simulink model "mech_gears_backlash"  (Simulink 7.1)
settings: Solver=ode23tb  StartTime=0.0  StopTime=20
InitFcn:
  | gear.backlashCW=0.2;
  | gear.backlashCCW=0.2;
undefined symbols (not defined in the file or in its folder): rad, s
libraries: mblibv1 x19, simulink x1
Description:
  | Gears with Backlash
  | 
  | Two gears with forward actuation and intergear backlash. Gear radius ratio: GearB:GearA is 1:3.
settings Model: Creator=arnav  LastModifiedBy=batserve  ExtModeAutoUpdateStatusClock=off
settings DataIOCC: OutputOption=SpecifiedOutputTimes  OutputTimes=linspace(0,20,300)  Refine=5
settings OptimizationCC: InlineInvariantSignals=on
settings DebuggingCC: SaveWithParameterizedLinksMsg=none  SignalResolutionControl=TryResolveAllWithWarning  SolverPrmCheckMsg=none  MultiTaskDSMMsg=warning  MultiTaskCondExecSysMsg=none  SigSpecEnsureSampleTimeMsg=none  StrictBusMsg=None
settings HardwareCC: TargetBitPerLong=64  TargetEndianess=LittleEndian  TargetWordSize=64  TargetHWDeviceType=MATLAB Host  ProdEqTarget=off
settings RTWCC: SystemTargetFile=rsim.tlc  TemplateMakefile=rsim_default_tmf  Description=Rapid Simulation Target  ProcessScript=rsim_make_rtw_hook  IncludeERTFirstTime=on
settings RSimTargetCC: TargetFcnLib=ansi_tfl_tmw.mat  TargetFunctionLibrary=ANSI_C  IsPILTarget=off  EnableShiftOperators=on  PortableWordSizes=off
settings SimMechanicsCC: VisOnUpdateDiagram=on  VisDuringSimulation=on  VisConfigFile=mech_gears_backlash.mat

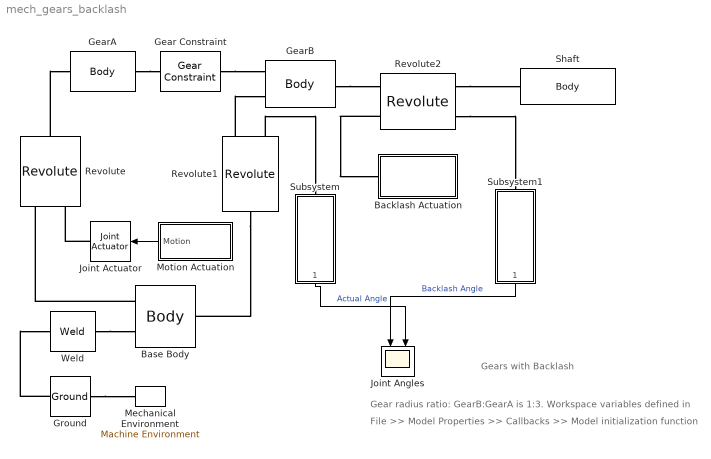
== system mech_gears_backlash ==
  note: Gears with Backlash
  note: Gear radius ratio: GearB:GearA is 1:3.
      | Workspace variables defined in
  note: File >> Model Properties >>
      | Callbacks >> Model initialization function
  Backlash Actuation : Subsystem
  Base Body : mblibv1/Bodies/Body  DialogController=MECH.DynMechDlgSource  PhysicalDomain=mechanical  SubClassName=Unknown  LeftPortType=workingframe  RightPortType=workingframe  LConnTagsString=CS1|CG  RConnTagsString=CS2  DialogClass=MechanicalBodyBlock  Mass=14  MassUnits=kg  InertiaUnits=kg*m^2  Inertia=[1 0 0;0 3 0;0 0 3];  Shape=Cylinder  ShapeDims=[1 1]  ShapeUnits=m  ShapeUse=false  Density=1  DensityUnits=kg/m^3  DensityUse=false  GraphicsMode=1  BodyColor=[0.5 0.5 0.5]  GraphicsObj=[]  AttachedToCS=1  CG=Left$CG$[1 0 0]$CS1$CS1$m$[0 0 0]$Euler X-Y-Z$deg$WORLD$true  WorkingFrames=Left$CS1$[0 0 0]$WORLD$WORLD$m$[0 0 0]$Euler X-Y-Z$deg$WORLD$true#Right$CS2$[2 0 0]$CS1$CS1$m$[0 0 0]$Euler X-Y-Z$deg$WORLD$true#Right$CS3$[1 -2 0]$CS1$CS1$m$[0 0 0]$Euler X-Y-Z$deg$WORLD$false  CGPos=[1 0 0]  CGRot=[0 0 0]  CS0Pos=[]  CS0Rot=[]  CS1Pos=[0 0 0]  CS1Rot=[0 0 0]  CS2Pos=[2 0 0]  CS2Rot=[0 0 0]  CS3Pos=[1 -2 0]  CS3Rot=[0 0 0]  CS4Pos=[]  CS4Rot=[]  CS5Pos=[]  CS5Rot=[]  CS6Pos=[]  CS6Rot=[]  CS7Pos=[]  CS7Rot=[]  CS8Pos=[]  CS8Rot=[]  CS9Pos=[]  CS9Rot=[]  CS10Pos=[]  CS10Rot=[]  CS11Pos=[]  CS11Rot=[]  CS12Pos=[]  CS12Rot=[]  CS13Pos=[]  CS13Rot=[]  CS14Pos=[]  CS14Rot=[]  CS15Pos=[]  CS15Rot=[]  CS16Pos=[]  CS16Rot=[]  CS17Pos=[]  CS17Rot=[]  CS18Pos=[]  CS18Rot=[]  CS19Pos=[]  CS19Rot=[]  CS20Pos=[]  CS20Rot=[]
  Gear Constraint : mblibv1/Constraints &  Drivers/Gear Constraint  DialogController=MECH.DynMechDlgSource  PhysicalDomain=mechanical  SubClassName=Unknown  LeftPortType=blob  RightPortType=blob  LConnTagsString=__newl0  RConnTagsString=__newr0  DialogClass=GearConstraint  NumSAPorts=0  BaseRadius=1.5  BaseRadiusUnits=m  FollowerRadius=0.5  FollowerRadiusUnits=m
  GearA : mblibv1/Bodies/Body  DialogController=MECH.DynMechDlgSource  PhysicalDomain=mechanical  SubClassName=Unknown  LeftPortType=workingframe  RightPortType=workingframe  LConnTagsString=CS1  RConnTagsString=CS2  DialogClass=MechanicalBodyBlock  Mass=2  MassUnits=kg  InertiaUnits=kg*m^2  Inertia=[0.5 0 0;0 0.5 0;0 0 1]  Shape=Cylinder  ShapeDims=[1 1]  ShapeUnits=m  ShapeUse=false  Density=1  DensityUnits=kg/m^3  DensityUse=false  GraphicsMode=1  BodyColor=[0.5 0.5 0.5]  GraphicsObj=[]  AttachedToCS=1  CG=Left$CG$[0 0 0]$CS1$CS1$m$[0 0 0]$Euler X-Y-Z$deg$WORLD$false  WorkingFrames=Left$CS1$[0 0 0]$ADJOINING$ADJOINING$m$[0 0 0]$Euler X-Y-Z$deg$WORLD$true#Right$CS2$[0 0 0]$CS1$CS1$m$[0 0 0]$Euler X-Y-Z$deg$WORLD$true#Right$CS3$[-1 0 0]$CG$CG$m$[0 0 0]$Euler X-Y-Z$deg$WORLD$false#Right$CS4$[0 1 0]$CG$CG$m$[0 0 0]$Euler X-Y-Z$deg$WORLD$false#Right$CS5$[1 0 0]$CG$CG$m$[0 0 0]$Euler X-Y-Z$deg$WORLD$false#Right$CS6$[0 -1 0]$CG$CG$m$[0 0 0]$Euler X-Y-Z$deg$WORLD$false#Right$CS7$[0 0 -0.5]$CS3$CS3$m$[0 0 0]$Euler X-Y-Z$deg$WORLD$false#Right$CS8$[0 0 -0.5]$CS4$CS4$m$[0 0 0]$Euler X-Y-Z$deg$WORLD$false#Right$CS9$[0 0 -0.5]$CS5$CS5$m$[0 0 0]$Euler X-Y-Z$deg$WORLD$false#Right$CS10$[0 0 -0.5]$CS6$CS6$m$[0 0 0]$Euler X-Y-Z$deg$WORLD$false  CGPos=[0 0 0]  CGRot=[0 0 0]  CS0Pos=[]  CS0Rot=[]  CS1Pos=[0 0 0]  CS1Rot=[0 0 0]  CS2Pos=[0 0 0]  CS2Rot=[0 0 0]  CS3Pos=[-1 0 0]  CS3Rot=[0 0 0]  CS4Pos=[0 1 0]  CS4Rot=[0 0 0]  CS5Pos=[1 0 0]  CS5Rot=[0 0 0]  CS6Pos=[0 -1 0]  CS6Rot=[0 0 0]  CS7Pos=[0 0 -0.5]  CS7Rot=[0 0 0]  CS8Pos=[0 0 -0.5]  CS8Rot=[0 0 0]  CS9Pos=[0 0 -0.5]  CS9Rot=[0 0 0]  CS10Pos=[0 0 -0.5]  CS10Rot=[0 0 0]  CS11Pos=[]  CS11Rot=[]  CS12Pos=[]  CS12Rot=[]  CS13Pos=[]  CS13Rot=[]  CS14Pos=[]  CS14Rot=[]  CS15Pos=[]  CS15Rot=[]  CS16Pos=[]  CS16Rot=[]  CS17Pos=[]  CS17Rot=[]  CS18Pos=[]  CS18Rot=[]  CS19Pos=[]  CS19Rot=[]  CS20Pos=[]  CS20Rot=[]
  GearB : mblibv1/Bodies/Body  DialogController=MECH.DynMechDlgSource  PhysicalDomain=mechanical  SubClassName=Unknown  LeftPortType=workingframe  RightPortType=workingframe  LConnTagsString=CS1|CS2  RConnTagsString=CS3  DialogClass=MechanicalBodyBlock  Mass=4  MassUnits=kg  InertiaUnits=kg*m^2  Inertia=[0.5 0 0;0 0.5 0;0 0 1]  Shape=Cylinder  ShapeDims=[1 1]  ShapeUnits=m  ShapeUse=false  Density=1  DensityUnits=kg/m^3  DensityUse=false  GraphicsMode=1  BodyColor=[0.5 0.5 0.5]  GraphicsObj=[]  AttachedToCS=1  CG=Left$CG$[0 0 0]$CS1$CS1$m$[0 0 0]$Euler X-Y-Z$deg$WORLD$false  WorkingFrames=Left$CS1$[2 0 0]$ADJOINING$ADJOINING$m$[0 0 0]$Euler X-Y-Z$deg$WORLD$true#Left$CS2$[0 0 0]$CS1$CS1$m$[0 0 0]$Euler X-Y-Z$deg$WORLD$true#Right$CS3$[0 0 0]$CS1$CS1$m$[0 0 0]$Euler X-Y-Z$deg$WORLD$true#Right$CS4$[1 0 0]$CG$CG$m$[0 0 0]$Euler X-Y-Z$deg$WORLD$false#Right$CS5$[0 1 0]$CG$CG$m$[0 0 0]$Euler X-Y-Z$deg$WORLD$false#Right$CS6$[-1 0 0]$CG$CG$m$[0 0 0]$Euler X-Y-Z$deg$WORLD$false#Right$CS7$[0 -1 0]$CG$CG$m$[0 0 0]$Euler X-Y-Z$deg$WORLD$false#Right$CS8$[0 0 -0.5]$CS4$CS4$m$[0 0 0]$Euler X-Y-Z$deg$WORLD$false#Right$CS9$[0 0 -0.5]$CS5$CS5$m$[0 0 0]$Euler X-Y-Z$deg$WORLD$false#Right$CS10$[0 0 -0.5]$CS6$CS6$m$[0 0 0]$Euler X-Y-Z$deg$WORLD$false#Right$CS11$[0 0 -0.5]$CS7$CS7$m$[0 0 0]$Euler X-Y-Z$deg$WORLD$false  CGPos=[0 0 0]  CGRot=[0 0 0]  CS0Pos=[]  CS0Rot=[]  CS1Pos=[2 0 0]  CS1Rot=[0 0 0]  CS2Pos=[0 0 0]  CS2Rot=[0 0 0]  CS3Pos=[0 0 0]  CS3Rot=[0 0 0]  CS4Pos=[1 0 0]  CS4Rot=[0 0 0]  CS5Pos=[0 1 0]  CS5Rot=[0 0 0]  CS6Pos=[-1 0 0]  CS6Rot=[0 0 0]  CS7Pos=[0 -1 0]  CS7Rot=[0 0 0]  CS8Pos=[0 0 -0.5]  CS8Rot=[0 0 0]  CS9Pos=[0 0 -0.5]  CS9Rot=[0 0 0]  CS10Pos=[0 0 -0.5]  CS10Rot=[0 0 0]  CS11Pos=[0 0 -0.5]  CS11Rot=[0 0 0]  CS12Pos=[]  CS12Rot=[]  CS13Pos=[]  CS13Rot=[]  CS14Pos=[]  CS14Rot=[]  CS15Pos=[]  CS15Rot=[]  CS16Pos=[]  CS16Rot=[]  CS17Pos=[]  CS17Rot=[]  CS18Pos=[]  CS18Rot=[]  CS19Pos=[]  CS19Rot=[]  CS20Pos=[]  CS20Rot=[]
  Ground : mblibv1/Bodies/Ground  Orientation=left  DialogController=MECH.DynMechDlgSource  SystemSampleTime=-1  LeftPortType=env  RightPortType=workingframe  PhysicalDomain=Mechanical  DialogClass=GroundBlock  CoordPosition=[1 0 0]  CoordPositionUnits=m  StateVectorMgrId=-1  MachineId=[0 0]  ShowEnvPort=on
  Joint Actuator : mblibv1/Sensors &  Actuators/Joint Actuator  Orientation=left  DialogController=MECH.DynMechDlgSource  SystemSampleTime=-1  PhysicalDomain=Mechanical  PortType=blob  ActuationStyle=Motion  AngleUnits=rad  ArcVelocityUnits=rad/s  ArcAccelerationUnits=rad/s^2  CoordPositionUnits=m  VelocityUnits=m/s  AccelerationUnits=m/s^2  ForceUnits=N  TorqueUnits=N-m  ActiveIO=on  Width=3  DialogClass=MechanicalActuatorBlock  Primitive=R1  ReferenceFrame=Absolute (INERTIAL)
  Joint Angles : Scope  NumInputPorts=2
      settings: Orientation=down  TimeRange=20  YMin=-0.25~-2  YMax=0.25~16  SaveName=ScopeData2
  Mechanical Environment : mblibv1/Bodies/Machine Environment  Tag=Factory ground  Orientation=left  DialogController=MECH.DialogSource  SystemSampleTime=-1  PortType=env  PhysicalDomain=Mechanical  DialogTemplateClass=MECH.MachineEnvironment  SyncWhenCopied=off  Gravity=[0 -9.81 0]  GravityUnits=m/s^2  GravityAsSignal=off  Dimensionality=3D Only  AnalysisType=Forward dynamics  LinearAssemblyTolerance=1e-3  LinearAssemblyToleranceUnits=m  AngularAssemblyTolerance=1e-3  AngularAssemblyToleranceUnits=rad  ConstraintSolverType=Stabilizing  ConstraintRelTolerance=1e-4  ConstraintAbsTolerance=1e-4  UseRobustSingularityHandling=off  RedundancyAnalysisToleranceType=Automatically select tolerance  RedundancyAnalysisTolerance=1e-14  StatePerturbationType=Fixed  PerturbationSize=1e-5  VisualizeMachine=on
  Motion Actuation : Subsystem  Orientation=left
  Revolute : mblibv1/Joints/Revolute  Orientation=up  DialogController=MECH.DynMechDlgSource  PhysicalDomain=mechanical  SubClassName=Unknown  LeftPortType=blob  RightPortType=blob  LConnTagsString=__newl0|SA1  RConnTagsString=__newr0  NumSAPorts=1  CutJoint=off  MarkAsCut=off  Primitives=revolute  PrimitiveProps=R1$WORLD$[0 0 1]$revolute  DialogClass=JointBlock  R1Axis=[0 0 1]
  Revolute1 : mblibv1/Joints/Revolute  Orientation=down  DialogController=MECH.DynMechDlgSource  PhysicalDomain=mechanical  SubClassName=Unknown  LeftPortType=blob  RightPortType=blob  LConnTagsString=__newl0|SA1  RConnTagsString=__newr0  NumSAPorts=1  CutJoint=off  MarkAsCut=off  Primitives=revolute  PrimitiveProps=R1$WORLD$[0 0 1]$revolute  DialogClass=JointBlock  R1Axis=[0 0 1]
  Revolute2 : mblibv1/Joints/Revolute  DialogController=MECH.DynMechDlgSource  PhysicalDomain=mechanical  SubClassName=Unknown  LeftPortType=blob  RightPortType=blob  LConnTagsString=__newl0|SA1  RConnTagsString=__newr0|SA1  NumSAPorts=2  CutJoint=off  MarkAsCut=off  Primitives=revolute  PrimitiveProps=R1$WORLD$[0 0 1]$revolute  DialogClass=JointBlock  R1Axis=[0 0 1]
  Shaft : mblibv1/Bodies/Body  DialogController=MECH.DynMechDlgSource  PhysicalDomain=mechanical  SubClassName=Unknown  LeftPortType=workingframe  RightPortType=workingframe  LConnTagsString=CS1  DialogClass=MechanicalBodyBlock  Mass=10  MassUnits=kg  InertiaUnits=kg*m^2  Inertia=[3 0 0;0 3 0;0 0 0.2];  Shape=Cylinder  ShapeDims=[1 1]  ShapeUnits=m  ShapeUse=false  Density=1  DensityUnits=kg/m^3  DensityUse=false  GraphicsMode=1  BodyColor=[0.5 0.5 0.5]  GraphicsObj=[]  AttachedToCS=1  CG=Left$CG$[0 0 1.5]$CS1$CS1$m$[0 0 0]$Euler X-Y-Z$deg$WORLD$false  WorkingFrames=Left$CS1$[0 0 0]$ADJOINING$ADJOINING$m$[0 0 0]$Euler X-Y-Z$deg$WORLD$true#Right$CS2$[0 1.5 0]$CG$CG$m$[0 0 0]$Euler X-Y-Z$deg$WORLD$false#Right$CS3$[0 -1.5 0]$CG$CG$m$[0 0 0]$Euler X-Y-Z$deg$WORLD$false#Right$CS4$[0 0 1]$CS2$CS2$m$[0 0 0]$Euler X-Y-Z$deg$WORLD$false#Right$CS5$[0 0 1]$CS3$CS3$m$[0 0 0]$Euler X-Y-Z$deg$WORLD$false  CGPos=[0 0 1.5]  CGRot=[0 0 0]  CS0Pos=[]  CS0Rot=[]  CS1Pos=[0 0 0]  CS1Rot=[0 0 0]  CS2Pos=[0 1.5 0]  CS2Rot=[0 0 0]  CS3Pos=[0 -1.5 0]  CS3Rot=[0 0 0]  CS4Pos=[0 0 1]  CS4Rot=[0 0 0]  CS5Pos=[0 0 1]  CS5Rot=[0 0 0]  CS6Pos=[]  CS6Rot=[]  CS7Pos=[]  CS7Rot=[]  CS8Pos=[]  CS8Rot=[]  CS9Pos=[]  CS9Rot=[]  CS10Pos=[]  CS10Rot=[]  CS11Pos=[]  CS11Rot=[]  CS12Pos=[]  CS12Rot=[]  CS13Pos=[]  CS13Rot=[]  CS14Pos=[]  CS14Rot=[]  CS15Pos=[]  CS15Rot=[]  CS16Pos=[]  CS16Rot=[]  CS17Pos=[]  CS17Rot=[]  CS18Pos=[]  CS18Rot=[]  CS19Pos=[]  CS19Rot=[]  CS20Pos=[]  CS20Rot=[]
  Subsystem : Subsystem  Orientation=down
  Subsystem1 : Subsystem  Orientation=down
  Weld : mblibv1/Joints/Weld  DialogController=MECH.DynMechDlgSource  PhysicalDomain=mechanical  SubClassName=Unknown  LeftPortType=blob  RightPortType=blob  LConnTagsString=__newl0  RConnTagsString=__newr0  NumSAPorts=0  CutJoint=off  MarkAsCut=off  Primitives=weld  PrimitiveProps=W$INERTIAL$[0 0 0]$weld  DialogClass=JointBlock  WAxis=[0 0 0]
  wires:
  Motion Actuation/1(Motion) -> Joint Actuator/1
  Subsystem1/1(Backlash Angle) -> Joint Angles/1  "Backlash Angle"
  Subsystem/1(Actual Angle) -> Joint Angles/2  "Actual Angle"
  connections:
  Gear Constraint/RConn1 -- GearB/LConn1
  GearA/RConn1 -- Gear Constraint/LConn1
  Ground/LConn1 -- Mechanical Environment/RConn1
  Revolute1/RConn1 -- Base Body/RConn1
  GearB/RConn1 -- Revolute2/LConn1
  Revolute2/RConn1 -- Shaft/LConn1
  Revolute1/LConn1 -- GearB/LConn2
  Ground/RConn1 -- Weld/LConn1
  Weld/RConn1 -- Base Body/LConn2
  Base Body/LConn1 -- Revolute/LConn1
  Revolute/RConn1 -- GearA/LConn1
  Joint Actuator/RConn1 -- Revolute/LConn2
  Revolute2/LConn2 -- Backlash Actuation/LConn1
  Revolute2/RConn2 -- Subsystem1/LConn1
  Revolute1/LConn2 -- Subsystem/LConn1

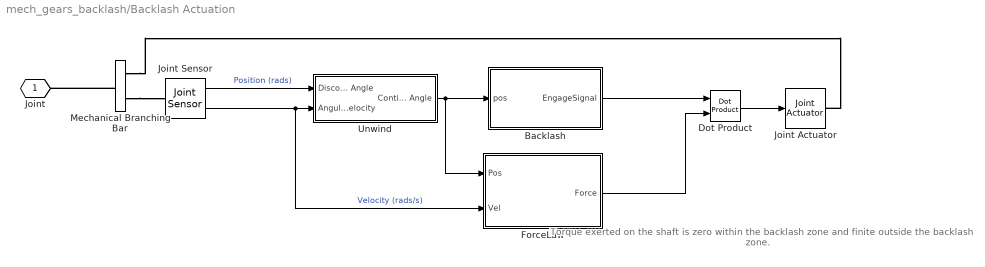
== system mech_gears_backlash/Backlash Actuation ==
  note: Torque exerted on the shaft is zero
      | within the backlash zone and finite
      | outside the backlash zone.
  Backlash : Subsystem
  Dot Product : simulink/Math Operations/Dot Product  InputSameDT=on  OutDataType=sfix(16)  OutScaling=2^-10  DoSatur=off
  ForceLaw : Subsystem
  Joint Actuator : mblibv1/Sensors &  Actuators/Joint Actuator  DialogController=MECH.DynMechDlgSource  SystemSampleTime=-1  PhysicalDomain=Mechanical  PortType=blob  ActuationStyle=Force  AngleUnits=deg  ArcVelocityUnits=deg/s  ArcAccelerationUnits=deg/s^2  CoordPositionUnits=m  VelocityUnits=m/s  AccelerationUnits=m/s^2  ForceUnits=N  TorqueUnits=N-m  ActiveIO=on  Width=1  DialogClass=MechanicalActuatorBlock  Primitive=R1  ReferenceFrame=Absolute (INERTIAL)
  Joint Sensor : mblibv1/Sensors &  Actuators/Joint Sensor  DialogController=MECH.DynMechDlgSource  SystemSampleTime=-1  PhysicalDomain=Mechanical  PortType=blob  Muxed=off  Pose=off  Angle=on  AngleUnits=rad  ArcVelocity=on  ArcVelocityUnits=rad/s  ArcAcceleration=off  ArcAccelerationUnits=deg/s^2  CoordPosition=off  CoordPositionUnits=m  Velocity=off  VelocityUnits=m/s  Acceleration=off  AccelerationUnits=m/s^2  Quaternion=off  QuaternionDT=off  QuaternionDDT=off  QuaternionUnits=off  OutputVector=[ 1 1 ]  ActiveIO=on  Width=2  DialogClass=MechanicalSensorBlock  Primitive=R1  Force=off  ForceUnits=N  Torque=off  TorqueUnits=N-m  ReferenceFrame=Absolute (INERTIAL)  ReactionSensedSide=Base  ReactionReferenceFrame=Absolute (World)  ReactionForce=off  ReactionForceUnits=N  ReactionMoment=off  ReactionMomentUnits=N-m
  Mechanical Branching Bar : mblibv1/Utilities/Mechanical Branching Bar  DialogController=MECH.DynMechDlgSource  PhysicalDomain=mechanical  SubClassName=Unknown  LeftPortType=blob  RightPortType=blob  LConnTagsString=_newl0  RConnTagsString=SA0|SA1  DialogClass=MechanicalBranchingBarBlock  NumSAPorts=2
  Unwind : Subsystem
  Joint : PMIOPort  Tag=PMCPort  Port=1  Side=Left
  wires:
  ForceLaw/1(Force) -> Dot Product/2
  Dot Product/1 -> Joint Actuator/1
  Backlash/1(EngageSignal) -> Dot Product/1
  Unwind/1(Continuous Angle) -> ForceLaw/1(Pos), Backlash/1(pos)
  Joint Sensor/1 -> Unwind/1(Discontinuous Angle)  "Position (rads)"
  Joint Sensor/2 -> ForceLaw/2(Vel), Unwind/2(Angular velocity)  "Velocity (rads/s)"
  connections:
  Mechanical Branching Bar/RConn1 -- Joint Actuator/RConn1
  Mechanical Branching Bar/RConn2 -- Joint Sensor/LConn1
  Mechanical Branching Bar/LConn1 -- Joint/RConn1

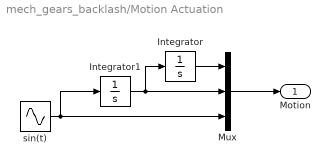
== system mech_gears_backlash/Motion Actuation ==
  Integrator : Integrator
  Integrator1 : Integrator  InitialCondition=-0.25
  Mux : Mux  Inputs=3
  sin(t) : Sin  Amplitude=0.5  SampleTime=0
  Motion : Outport  OutDataType=sfix(16)  OutScaling=2^0
  wires:
  Integrator1/1 -> Mux/2, Integrator/1
  sin(t)/1 -> Integrator1/1, Mux/3
  Mux/1 -> Motion/1
  Integrator/1 -> Mux/1

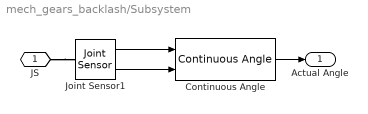
== system mech_gears_backlash/Subsystem ==
  Continuous Angle : mblibv1/Utilities/Continuous Angle  Tag=Factory continuousAngle  SystemSampleTime=-1  rad=rad  rads=rad/s
  Joint Sensor1 : mblibv1/Sensors &  Actuators/Joint Sensor  DialogController=MECH.DynMechDlgSource  SystemSampleTime=-1  PhysicalDomain=Mechanical  PortType=blob  Muxed=off  Pose=off  Angle=on  AngleUnits=rad  ArcVelocity=on  ArcVelocityUnits=rad/s  ArcAcceleration=off  ArcAccelerationUnits=deg/s^2  CoordPosition=on  CoordPositionUnits=m  Velocity=off  VelocityUnits=m/s  Acceleration=off  AccelerationUnits=m/s^2  Quaternion=on  QuaternionDT=off  QuaternionDDT=off  QuaternionUnits=off  OutputVector=[ 1 1 ]  ActiveIO=on  Width=2  DialogClass=MechanicalSensorBlock  Primitive=R1  Force=off  ForceUnits=N  Torque=off  TorqueUnits=N-m  ReferenceFrame=Absolute (INERTIAL)  ReactionSensedSide=Base  ReactionReferenceFrame=Absolute (World)  ReactionForce=off  ReactionForceUnits=N  ReactionMoment=off  ReactionMomentUnits=N-m
  JS : PMIOPort  Port=1  Side=Left
  Actual Angle : Outport  OutDataType=sfix(16)  OutScaling=2^0
  wires:
  Joint Sensor1/2 -> Continuous Angle/2
  Joint Sensor1/1 -> Continuous Angle/1
  Continuous Angle/1 -> Actual Angle/1
  connections:
  JS/RConn1 -- Joint Sensor1/LConn1

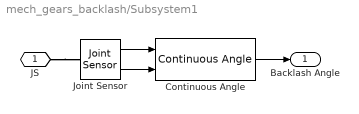
== system mech_gears_backlash/Subsystem1 ==
  Continuous Angle : mblibv1/Utilities/Continuous Angle  Tag=Factory continuousAngle  SystemSampleTime=-1  rad=rad  rads=rad/s
  Joint Sensor : mblibv1/Sensors &  Actuators/Joint Sensor  DialogController=MECH.DynMechDlgSource  SystemSampleTime=-1  PhysicalDomain=Mechanical  PortType=blob  Muxed=off  Pose=off  Angle=on  AngleUnits=rad  ArcVelocity=on  ArcVelocityUnits=rad/s  ArcAcceleration=off  ArcAccelerationUnits=deg/s^2  CoordPosition=on  CoordPositionUnits=m  Velocity=off  VelocityUnits=m/s  Acceleration=off  AccelerationUnits=m/s^2  Quaternion=on  QuaternionDT=off  QuaternionDDT=off  QuaternionUnits=off  OutputVector=[ 1 1 ]  ActiveIO=on  Width=2  DialogClass=MechanicalSensorBlock  Primitive=R1  Force=off  ForceUnits=N  Torque=off  TorqueUnits=N-m  ReferenceFrame=Absolute (INERTIAL)  ReactionSensedSide=Base  ReactionReferenceFrame=Absolute (World)  ReactionForce=off  ReactionForceUnits=N  ReactionMoment=off  ReactionMomentUnits=N-m
  JS : PMIOPort  Port=1  Side=Left
  Backlash Angle : Outport  OutDataType=sfix(16)  OutScaling=2^0
  wires:
  Continuous Angle/1 -> Backlash Angle/1
  Joint Sensor/2 -> Continuous Angle/2
  Joint Sensor/1 -> Continuous Angle/1
  connections:
  JS/RConn1 -- Joint Sensor/LConn1

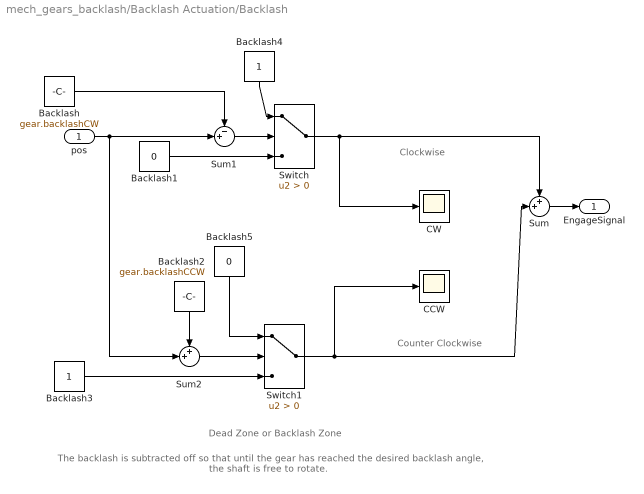
== system mech_gears_backlash/Backlash Actuation/Backlash ==
  note: The backlash is subtracted off so that until the gear
      | has reached the desired backlash angle, the shaft is free to rotate.
  note: Dead Zone or Backlash Zone
  note: Counter Clockwise
  note: Clockwise
  pos : Inport  OutDataType=sfix(16)  OutScaling=2^0
  Backlash : Constant  Value=gear.backlashCW  OutDataType=sfix(16)  OutScaling=2^0
  Backlash1 : Constant  Value=0  OutDataType=sfix(16)  OutScaling=2^0
  Backlash2 : Constant  Orientation=down  Value=gear.backlashCCW  OutDataType=sfix(16)  OutScaling=2^0
  Backlash3 : Constant  OutDataType=sfix(16)  OutScaling=2^0
  Backlash4 : Constant  Orientation=down  OutDataType=sfix(16)  OutScaling=2^0
  Backlash5 : Constant  Orientation=down  Value=0  OutDataType=sfix(16)  OutScaling=2^0
  CCW : Scope
      settings: TimeRange=5  YMin=-4  YMax=2.5  SaveName=ScopeData4
  CW : Scope
      settings: TimeRange=5  YMin=0  YMax=1
  Sum : Sum  Inputs=++|  OutDataType=sfix(16)  OutScaling=2^0  SaturateOnIntegerOverflow=on
  Sum1 : Sum  Inputs=-+|  OutDataType=sfix(16)  OutScaling=2^0  SaturateOnIntegerOverflow=on
  Sum2 : Sum  Inputs=++|  OutDataType=sfix(16)  OutScaling=2^0  SaturateOnIntegerOverflow=on
  Switch : Switch  Criteria=u2 > Threshold
  Switch1 : Switch  Criteria=u2 > Threshold
  EngageSignal : Outport  OutDataType=sfix(16)  OutScaling=2^0
  wires:
  Backlash5/1 -> Switch1/1
  Switch1/1 -> Sum/2, CCW/1
  Switch/1 -> CW/1, Sum/1
  Backlash4/1 -> Switch/1
  Sum/1 -> EngageSignal/1
  Backlash3/1 -> Switch1/3
  Sum2/1 -> Switch1/2
  Backlash2/1 -> Sum2/1
  Backlash1/1 -> Switch/3
  Sum1/1 -> Switch/2
  Backlash/1 -> Sum1/1
  pos/1 -> Sum2/2, Sum1/2

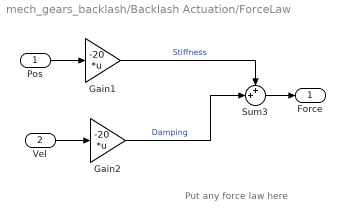
== system mech_gears_backlash/Backlash Actuation/ForceLaw ==
  note: Put any force law here
  Pos : Inport  OutDataType=sfix(16)  OutScaling=2^0
  Vel : Inport  Port=2  OutDataType=sfix(16)  OutScaling=2^0
  Gain1 : Gain  Gain=-20  Multiplication=Matrix(K*u)  ParameterDataType=sfix(16)  ParameterScaling=2^0  OutDataType=sfix(16)  OutScaling=2^0  SaturateOnIntegerOverflow=on  OutDataTypeStr=Inherit: Same as input  ParamDataTypeStr=Inherit: Same as input
  Gain2 : Gain  Gain=-20  Multiplication=Matrix(K*u)  ParameterDataType=sfix(16)  ParameterScaling=2^0  OutDataType=sfix(16)  OutScaling=2^0  SaturateOnIntegerOverflow=on  OutDataTypeStr=Inherit: Same as input  ParamDataTypeStr=Inherit: Same as input
  Sum3 : Sum  Inputs=++|  OutDataType=sfix(16)  OutScaling=2^0  SaturateOnIntegerOverflow=on
  Force : Outport  OutDataType=sfix(16)  OutScaling=2^0
  wires:
  Sum3/1 -> Force/1
  Vel/1 -> Gain2/1
  Pos/1 -> Gain1/1
  Gain2/1 -> Sum3/2  "Damping"
  Gain1/1 -> Sum3/1  "Stiffness"

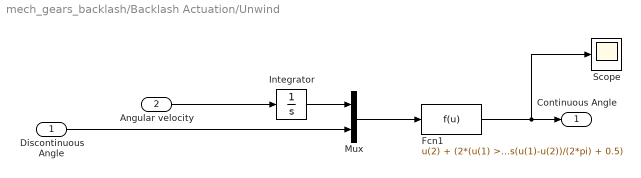
== system mech_gears_backlash/Backlash Actuation/Unwind ==
  Discontinuous Angle : Inport  OutDataType=sfix(16)  OutScaling=2^0
  Angular velocity : Inport  Port=2  OutDataType=sfix(16)  OutScaling=2^0
  Fcn1 : Fcn  Expr=u(2) + (2*(u(1) > u(2)) - 1)*2*pi*floor(abs(u(1)-u(2))/(2*pi) + 0.5)
  Integrator : Integrator  AbsoluteTolerance=1e-3
  Mux : Mux  Inputs=2
  Scope : Scope
  Continuous Angle : Outport  OutDataType=sfix(16)  OutScaling=2^0
  wires:
  Integrator/1 -> Mux/1
  Mux/1 -> Fcn1/1
  Fcn1/1 -> Continuous Angle/1, Scope/1
  Angular velocity/1 -> Integrator/1
  Discontinuous Angle/1 -> Mux/2
